simulink model "DSP"  (R2016b)
settings: Solver=VariableStepAuto  StartTime=0.0  StopTime=10.0  RelTol=1e-3
libraries: dsparch4 x2, commchan3 x1, commrandsrc3 x1
settings Model: Creator=white  LastModifiedBy=white

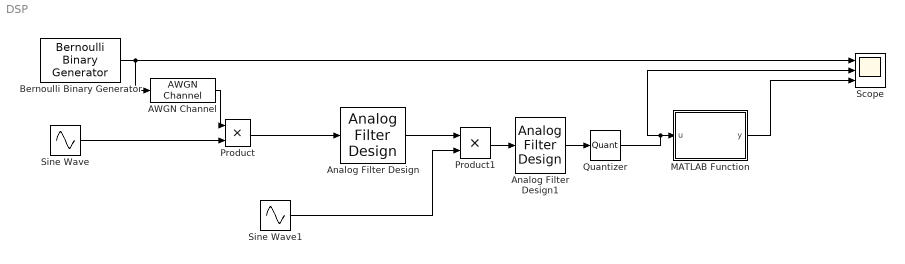
== system DSP ==
  AWGN Channel : commchan3/AWGN Channel  InputProcessing=Columns as channels (frame based)  seed=67  noiseMode="Signal to noise ratio  (Eb/No)"  EbNodB=10  EsNodB=10  SNRdB=20  bitsPerSym=1  Ps=1  Tsym=1  variance=1
  Analog Filter Design : dsparch4/Analog Filter Design  method=Butterworth  filttype=Bandpass  N=1  Wlo=98*2*pi  Whi=102*2*pi  Rp=2  Rs=40
  Analog Filter Design1 : dsparch4/Analog Filter Design  method=Butterworth  filttype=Lowpass  N=1  Wlo=4*pi  Whi=102*2*pi  Rp=2  Rs=40
  Bernoulli Binary Generator : commrandsrc3/Bernoulli Binary Generator  ProbabilityOfZero=0.5  SeedSource=Auto  Seed=0  SampleTime=1  SamplesPerFrame=1  OutputDataType=double  SimulateUsing=Interpreted execution
  MATLAB Function : MATLAB Function  TreatAsAtomicUnit=on
  Product : Product
  Product1 : Product
  Quantizer : Quantizer
  Scope : Scope  NumInputPorts=3
  Sine Wave : Sin  Frequency=100*2*pi  SampleTime=0.001
  Sine Wave1 : Sin  Frequency=100*2*pi  SampleTime=0.001
  wires:
  Sine Wave/1 -> Product/2
  Analog Filter Design/1 -> Product1/1
  Bernoulli Binary Generator/1 -> AWGN Channel/1, Scope/1
  Analog Filter Design1/1 -> Quantizer/1
  Quantizer/1 -> Scope/2, MATLAB Function/1(u)
  MATLAB Function/1(y) -> Scope/3
  Product1/1 -> Analog Filter Design1/1
  AWGN Channel/1 -> Product/1
  Product/1 -> Analog Filter Design/1
  Sine Wave1/1 -> Product1/2

== matlab function DSP/MATLAB Function ==
  data: u input; y output
function y = fcn(u)
if(u>0.25)
    u=1
else
    u=0
end
y = u;
